simulink model "FeedBack_Linearization"  (R2021b)
settings: Solver=VariableStepAuto  StartTime=0.0  StopTime=10.0  RelTol=1e-3
undefined symbols (not defined in the file): Kd, Kp, q_dq_init
(part 9 of 9)

== matlab function FeedBack_Linearization/G ==
  data: q input; G output; g input
function G = G_fun(q,g)
%G_fun
%    G = G_fun(Q1,Q2,Q3,Q4,Q5,Q6,Q7,g)

%    This function was generated by the Symbolic Math Toolbox version 9.0.
%    15-Apr-2022 03:01:31

q1 = q(1);
q2 = q(2);
q3 = q(3);
q4 = q(4);
q5 = q(5);
q6 = q(6);
q7 = q(7);



t2 = cos(q2);
t3 = cos(q3);
t4 = cos(q4);
t5 = cos(q5);
t6 = cos(q6);
t7 = cos(q7);
t8 = sin(q2);
t9 = sin(q3);
t10 = sin(q4);
t11 = sin(q5);
t12 = sin(q6);
t13 = sin(q7);
et1 = g.*t2.*3.45360925e-2-g.*t8.*4.3163130985+g.*t2.*t3.*5.5242e-3-g.*t2.*t9.*1.85444563e-1;
et2 = g.*t4.*t8.*(-2.002662146)-g.*t8.*t10.*5.2231e-4-g.*t2.*t3.*t4.*5.2231e-4+g.*t2.*t3.*t10.*2.002662146;
et3 = g.*t2.*t5.*t9.*(-1.01250325e-1)-g.*t4.*t6.*t8.*1.532971099999998e-3+g.*t2.*t9.*t11.*1.705e-4-g.*t5.*t8.*t10.*1.705e-4;
et4 = g.*t4.*t8.*t12.*1.6600955e-3-g.*t8.*t10.*t11.*1.01250325e-1-g.*t2.*t3.*t4.*t5.*1.705e-4-g.*t2.*t3.*t4.*t11.*1.01250325e-1;
et5 = g.*t2.*t3.*t6.*t10.*1.532971099999998e-3-g.*t2.*t5.*t7.*t9.*8.2343968e-3-g.*t2.*t3.*t10.*t12.*1.6600955e-3+g.*t2.*t6.*t9.*t11.*1.6600955e-3;
et6 = g.*t2.*t5.*t9.*t13.*(-1.22807312e-2)-g.*t5.*t6.*t8.*t10.*1.6600955e-3-g.*t4.*t7.*t8.*t12.*1.22807312e-2+g.*t2.*t9.*t11.*t12.*1.532971099999998e-3;
et7 = g.*t5.*t8.*t10.*t12.*(-1.532971099999998e-3)-g.*t7.*t8.*t10.*t11.*8.2343968e-3+g.*t4.*t8.*t12.*t13.*8.2343968e-3-g.*t8.*t10.*t11.*t13.*1.22807312e-2;
et8 = g.*t2.*t3.*t4.*t5.*t6.*(-1.6600955e-3)-g.*t2.*t3.*t4.*t5.*t12.*1.532971099999998e-3-g.*t2.*t3.*t4.*t7.*t11.*8.2343968e-3-g.*t2.*t3.*t4.*t11.*t13.*1.22807312e-2;
et9 = g.*t2.*t3.*t7.*t10.*t12.*1.22807312e-2-g.*t2.*t6.*t7.*t9.*t11.*1.22807312e-2+g.*t5.*t6.*t7.*t8.*t10.*1.22807312e-2-g.*t2.*t3.*t10.*t12.*t13.*8.2343968e-3;
et10 = g.*t2.*t6.*t9.*t11.*t13.*8.2343968e-3-g.*t5.*t6.*t8.*t10.*t13.*8.2343968e-3+g.*t2.*t3.*t4.*t5.*t6.*t7.*1.22807312e-2-g.*t2.*t3.*t4.*t5.*t6.*t13.*8.2343968e-3;
et11 = g.*t3.*t8.*(-1.85444563e-1)-g.*t8.*t9.*5.5242e-3-g.*t3.*t5.*t8.*1.01250325e-1+g.*t4.*t8.*t9.*5.2231e-4;
et12 = g.*t3.*t8.*t11.*1.705e-4-g.*t8.*t9.*t10.*2.002662146-g.*t3.*t5.*t7.*t8.*8.2343968e-3+g.*t4.*t5.*t8.*t9.*1.705e-4;
et13 = g.*t3.*t6.*t8.*t11.*1.6600955e-3-g.*t3.*t5.*t8.*t13.*1.22807312e-2+g.*t4.*t8.*t9.*t11.*1.01250325e-1-g.*t6.*t8.*t9.*t10.*1.532971099999998e-3;
et14 = g.*t3.*t8.*t11.*t12.*1.532971099999998e-3+g.*t8.*t9.*t10.*t12.*1.6600955e-3+g.*t4.*t5.*t6.*t8.*t9.*1.6600955e-3-g.*t3.*t6.*t7.*t8.*t11.*1.22807312e-2;
et15 = g.*t4.*t5.*t8.*t9.*t12.*1.532971099999998e-3+g.*t4.*t7.*t8.*t9.*t11.*8.2343968e-3+g.*t3.*t6.*t8.*t11.*t13.*8.2343968e-3+g.*t4.*t8.*t9.*t11.*t13.*1.22807312e-2;
et16 = g.*t7.*t8.*t9.*t10.*t12.*(-1.22807312e-2)+g.*t8.*t9.*t10.*t12.*t13.*8.2343968e-3-g.*t4.*t5.*t6.*t7.*t8.*t9.*1.22807312e-2+g.*t4.*t5.*t6.*t8.*t9.*t13.*8.2343968e-3;
et17 = g.*t2.*t4.*5.2231e-4-g.*t2.*t10.*2.002662146+g.*t2.*t4.*t5.*1.705e-4+g.*t3.*t4.*t8.*2.002662146;
et18 = g.*t2.*t4.*t11.*1.01250325e-1-g.*t2.*t6.*t10.*1.532971099999998e-3+g.*t3.*t8.*t10.*5.2231e-4+g.*t2.*t10.*t12.*1.6600955e-3;
et19 = g.*t2.*t4.*t5.*t6.*1.6600955e-3+g.*t3.*t4.*t6.*t8.*1.532971099999998e-3+g.*t2.*t4.*t5.*t12.*1.532971099999998e-3+g.*t2.*t4.*t7.*t11.*8.2343968e-3;
et20 = g.*t3.*t5.*t8.*t10.*1.705e-4-g.*t3.*t4.*t8.*t12.*1.6600955e-3+g.*t2.*t4.*t11.*t13.*1.22807312e-2-g.*t2.*t7.*t10.*t12.*1.22807312e-2;
et21 = g.*t3.*t8.*t10.*t11.*1.01250325e-1+g.*t2.*t10.*t12.*t13.*8.2343968e-3-g.*t2.*t4.*t5.*t6.*t7.*1.22807312e-2+g.*t2.*t4.*t5.*t6.*t13.*8.2343968e-3;
et22 = g.*t3.*t5.*t6.*t8.*t10.*1.6600955e-3+g.*t3.*t4.*t7.*t8.*t12.*1.22807312e-2+g.*t3.*t5.*t8.*t10.*t12.*1.532971099999998e-3+g.*t3.*t7.*t8.*t10.*t11.*8.2343968e-3;
et23 = g.*t3.*t4.*t8.*t12.*t13.*(-8.2343968e-3)+g.*t3.*t8.*t10.*t11.*t13.*1.22807312e-2-g.*t3.*t5.*t6.*t7.*t8.*t10.*1.22807312e-2+g.*t3.*t5.*t6.*t8.*t10.*t13.*8.2343968e-3;
et24 = g.*t2.*t5.*t10.*1.01250325e-1+g.*t5.*t8.*t9.*1.705e-4-g.*t2.*t10.*t11.*1.705e-4+g.*t8.*t9.*t11.*1.01250325e-1;
et25 = g.*t3.*t4.*t5.*t8.*(-1.01250325e-1)+g.*t2.*t5.*t7.*t10.*8.2343968e-3+g.*t3.*t4.*t8.*t11.*1.705e-4+g.*t5.*t6.*t8.*t9.*1.6600955e-3;
et26 = g.*t2.*t6.*t10.*t11.*(-1.6600955e-3)+g.*t2.*t5.*t10.*t13.*1.22807312e-2+g.*t5.*t8.*t9.*t12.*1.532971099999998e-3-g.*t2.*t10.*t11.*t12.*1.532971099999998e-3;
et27 = g.*t7.*t8.*t9.*t11.*8.2343968e-3+g.*t8.*t9.*t11.*t13.*1.22807312e-2-g.*t3.*t4.*t5.*t7.*t8.*8.2343968e-3+g.*t3.*t4.*t6.*t8.*t11.*1.6600955e-3;
et28 = g.*t3.*t4.*t5.*t8.*t13.*(-1.22807312e-2)-g.*t5.*t6.*t7.*t8.*t9.*1.22807312e-2+g.*t2.*t6.*t7.*t10.*t11.*1.22807312e-2+g.*t3.*t4.*t8.*t11.*t12.*1.532971099999998e-3;
et29 = g.*t5.*t6.*t8.*t9.*t13.*8.2343968e-3-g.*t2.*t6.*t10.*t11.*t13.*8.2343968e-3-g.*t3.*t4.*t6.*t7.*t8.*t11.*1.22807312e-2+g.*t3.*t4.*t6.*t8.*t11.*t13.*8.2343968e-3;
et30 = g.*t2.*t4.*t6.*(-1.6600955e-3)-g.*t2.*t4.*t12.*1.532971099999998e-3+g.*t2.*t4.*t6.*t7.*1.22807312e-2+g.*t2.*t5.*t6.*t10.*1.532971099999998e-3;
et31 = g.*t2.*t4.*t6.*t13.*(-8.2343968e-3)-g.*t3.*t6.*t8.*t10.*1.6600955e-3-g.*t2.*t5.*t10.*t12.*1.6600955e-3-g.*t3.*t8.*t10.*t12.*1.532971099999998e-3;
et32 = g.*t6.*t8.*t9.*t11.*1.532971099999998e-3-g.*t8.*t9.*t11.*t12.*1.6600955e-3-g.*t3.*t4.*t5.*t6.*t8.*1.532971099999998e-3+g.*t3.*t4.*t5.*t8.*t12.*1.6600955e-3;
et33 = g.*t3.*t6.*t7.*t8.*t10.*1.22807312e-2+g.*t2.*t5.*t7.*t10.*t12.*1.22807312e-2-g.*t3.*t6.*t8.*t10.*t13.*8.2343968e-3-g.*t2.*t5.*t10.*t12.*t13.*8.2343968e-3;
et34 = g.*t7.*t8.*t9.*t11.*t12.*1.22807312e-2-g.*t8.*t9.*t11.*t12.*t13.*8.2343968e-3-g.*t3.*t4.*t5.*t7.*t8.*t12.*1.22807312e-2+g.*t3.*t4.*t5.*t8.*t12.*t13.*8.2343968e-3;
et35 = g.*t2.*t4.*t7.*t12.*(-8.2343968e-3)-g.*t5.*t7.*t8.*t9.*1.22807312e-2+g.*t2.*t7.*t10.*t11.*1.22807312e-2-g.*t2.*t4.*t12.*t13.*1.22807312e-2;
et36 = g.*t5.*t8.*t9.*t13.*8.2343968e-3-g.*t2.*t10.*t11.*t13.*8.2343968e-3+g.*t2.*t5.*t6.*t7.*t10.*8.2343968e-3-g.*t3.*t4.*t7.*t8.*t11.*1.22807312e-2;
et37 = g.*t2.*t5.*t6.*t10.*t13.*1.22807312e-2+g.*t3.*t4.*t8.*t11.*t13.*8.2343968e-3-g.*t3.*t7.*t8.*t10.*t12.*8.2343968e-3+g.*t6.*t7.*t8.*t9.*t11.*8.2343968e-3;
et38 = g.*t3.*t8.*t10.*t12.*t13.*(-1.22807312e-2)+g.*t6.*t8.*t9.*t11.*t13.*1.22807312e-2-g.*t3.*t4.*t5.*t6.*t7.*t8.*8.2343968e-3-g.*t3.*t4.*t5.*t6.*t8.*t13.*1.22807312e-2;
G = [0.0;et1+et2+et3+et4+et5+et6+et7+et8+et9+et10;et11+et12+et13+et14+et15+et16;et17+et18+et19+et20+et21+et22+et23;et24+et25+et26+et27+et28+et29;et30+et31+et32+et33+et34;et35+et36+et37+et38];

== matlab function FeedBack_Linearization/Robot ==
  data: q_dq input; dq_ddq output; u input; q output; dq output; g input
function [dq_ddq,q,dq] = Robot(q_dq,u,g)
    q = q_dq(1:length(q_dq)/2);
    dq = q_dq(length(q_dq)/2+1:length(q_dq));
    g_num = g;


    M = M_fun(q);
    C = C_fun(q,dq);
    G = G_fun(q,g_num);

    ddq = M\(u - C - G);
    
    dq_ddq = [dq;ddq];

end
